simulink model "Potentiometer_Reader"  (R2024b)
settings: Solver=FixedStepAuto  StartTime=0.0  StopTime=inf  FixedStep=0.1  RelTol=1e-3  EnableMultiTasking=on
libraries: stm32f4xxblockslib x1
settings Model: STM32="{\"AnalogInput\":{\"ID\":\"Potentiometer_Reader:1\"}}"  Creator=Kaitniyom  LastModifiedBy=ACER
settings OptimizationCC: DefaultParameterBehavior=Inlined  EnhancedBackFolding=on  PassReuseOutputArgsAs=Individual arguments  ZeroExternalMemoryAtStartup=off  ZeroInternalMemoryAtStartup=off  MaxStackSize=512  OptimizeBlockOrder=speed  DifferentSizesBufferReuse=on  OptimizationCustomize=off  EfficientTunableParamExpr=on
settings DebuggingCC: ParameterTunabilityLossMsg=error
settings HardwareCC: ProdBitPerPointer=32  ProdBitPerSizeT=32  ProdBitPerPtrDiffT=32  ProdLargestAtomicInteger=Long  ProdLargestAtomicFloat=Double  ProdWordSize=32  ProdLongLongMode=on  ProdHWDeviceType=ARM Compatible->ARM Cortex-M
settings SFSimCC: MATLABDynamicMemAlloc=off
settings RTWCC: Description=Embedded Coder  SystemTargetFile=ert.tlc  HardwareBoard=STM32G4xx Based  TemplateMakefile=ert_default_tmf  Toolchain=GNU Tools for ARM Embedded Processors
settings CodeAppCC: ForceParamTrailComments=on  IgnoreCustomStorageClasses=off  OperatorAnnotations=on  SimulinkDataObjDesc=on  SFDataObjDesc=on  InsertBlockDesc=on
settings ERTTargetCC: TargetLangStandard=C99 (ISO)  CodeReplacementLibrary=ARM Cortex-M  ExtModeTransport=3  ExtModeStaticAlloc=on  ExtModeStaticAllocSize=2048  ExtModeMexFile=ext_xcp  ExtModeIntrfLevel=Level2 - Open

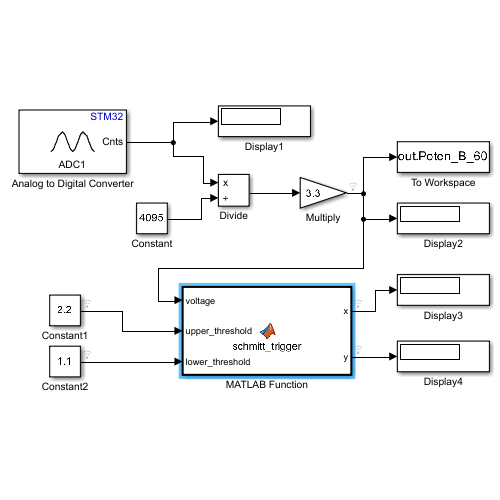
[thumbnail: Simulink's stored preview of the top-level diagram]
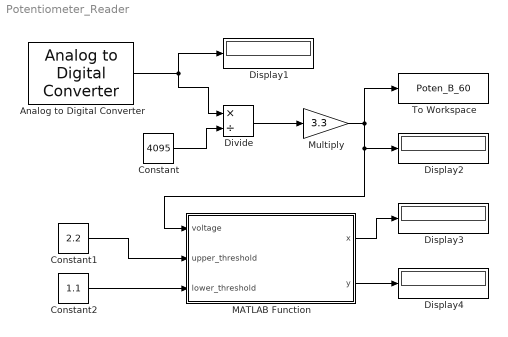
== system Potentiometer_Reader ==
  Analog to Digital Converter : stm32f4xxblockslib/Analog to Digital Converter  ADCModule=ADC1  ConversionGroup=Regular  TriggerMode=Trigger and read  NumberOfConversions=1  EnableBufferConv=off  BufferLength=1  OutputStatus=off  SampleTime=-1  EnableSimPort=off  hoistedMaskSrc=ECSoC/ECSimCodegen/Analog to Digital Converter
  Constant : Constant  Value=4095
  Constant1 : Constant  Value=2.2
  Constant2 : Constant  Value=1.1
  Display{1..4} (4 alike) : Display
  Divide : Product  Inputs=*/
  MATLAB Function : MATLAB Function  TreatAsAtomicUnit=on
  Multiply : Gain  Gain=3.3
  To Workspace : ToWorkspace  VariableName=Poten_B_60  SampleTime=-1
      settings: MaxDataPoints=100  Save2DSignal=2-D array (concatenate along first dimension)
  wires:
  Analog to Digital Converter/1 -> Divide/1, Display1/1
  Divide/1 -> Multiply/1
  Constant/1 -> Divide/2
  Multiply/1 -> MATLAB Function/1(voltage), Display2/1, To Workspace/1
  MATLAB Function/2(y) -> Display4/1
  Constant1/1 -> MATLAB Function/2(upper_threshold)
  Constant2/1 -> MATLAB Function/3(lower_threshold)
  MATLAB Function/1(x) -> Display3/1

== matlab function Potentiometer_Reader/MATLAB Function ==
  data: x output; voltage input; y output; upper_threshold input; lower_threshold input
function [x, y] = schmitt_trigger(voltage, upper_threshold, lower_threshold)
    % Persistent variable to store the output state
    persistent state1;
    persistent state2;

    % Initialize the state variable on the first run
    if isempty(state1)
        state1 = 0; % Initial output state
    end
    if isempty(state2)
        state2 = 0; % Initial output state
    end
    
    % Check the input signal against the thresholds
    if voltage > upper_threshold
        state1 = 1;
        state2 = 3.3; % Set the output to high
    elseif voltage < lower_threshold
        state1 = 0; % Set the output to low
        state2 = 0;
    end

    x = state1;
    y = state2;
end
